simulink model "buck_discrete_sw_Close_Caso_2"  (R2025a)
settings: Solver=FixedStepDiscrete  StartTime=0.0  StopTime=inf  FixedStep=Tsim  RelTol=RelativeTolerance  EnableMultiTasking=on
undefined symbols (not defined in the file or in its folder): C_buck, DiscIntNeverNeededParam, L_buck, R, Scaling_Current, Scaling_Voltage, Vg
libraries: c2837xDlib x3
settings Model: ExtModeTrigDuration=8  Creator=Fernand  LastModifiedBy=Andres
settings DataIOCC: SaveFormat=StructureWithTime  ReturnWorkspaceOutputs=off  OutputSaveName=data_results  SignalLoggingName=DataResult
settings OptimizationCC: DefaultUnderspecifiedDataType=single  EnhancedBackFolding=on  PassReuseOutputArgsAs=Individual arguments  MaxStackSize=1024  OptimizeBlockOrder=speed  DifferentSizesBufferReuse=on  OptimizationCustomize=off  EfficientTunableParamExpr=on
settings DebuggingCC: ArtificialAlgebraicLoopMsg=none  ParameterTunabilityLossMsg=error
settings HardwareCC: ProdBitPerChar=16.0  ProdBitPerInt=16.0  ProdBitPerPointer=32.0  ProdBitPerSizeT=32.0  ProdBitPerPtrDiffT=32.0  ProdLargestAtomicInteger=Integer  ProdLargestAtomicFloat=None  ProdWordSize=16.0  ProdLongLongMode=on  ProdHWDeviceType=Texas Instruments->C2000  HardwareBoardFeatureSet=SoCBlockset
settings ModelReferenceCC: ModelReferenceNumInstancesAllowed=Single
settings SFSimCC: MATLABDynamicMemAlloc=off
settings RTWCC: SystemTargetFile=ert.tlc  HardwareBoard=TI Delfino F28379D LaunchPad  TemplateMakefile=ert_default_tmf  Toolchain=Texas Instruments Code Composer Studio (C2000)  CodeProfilingSaveOptions=MetricsOnly  GPUComputeCapability=3.5  Description=Embedded Coder
settings CodeAppCC: ForceParamTrailComments=on  IgnoreCustomStorageClasses=off  OperatorAnnotations=on  SimulinkDataObjDesc=on  SFDataObjDesc=on  InsertBlockDesc=on
settings ERTTargetCC: ExtModeTransport=4.0  ExtModeAutomaticAllocSize=off  ExtModeStaticAllocSize=10000.0  InlinedParameterPlacement=Hierarchical  DynamicArrayContainerType=coder::array  CodeReplacementLibrary=TI C28x  SubcomponentCodeInterfacePackaging=Nonreusable function  SupportContinuousTime=on

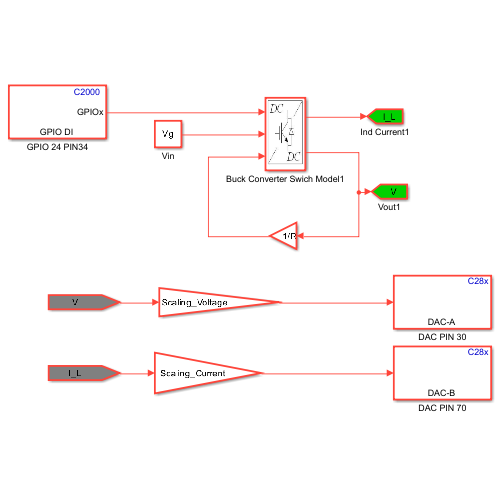
[thumbnail: Simulink's stored preview of the top-level diagram]
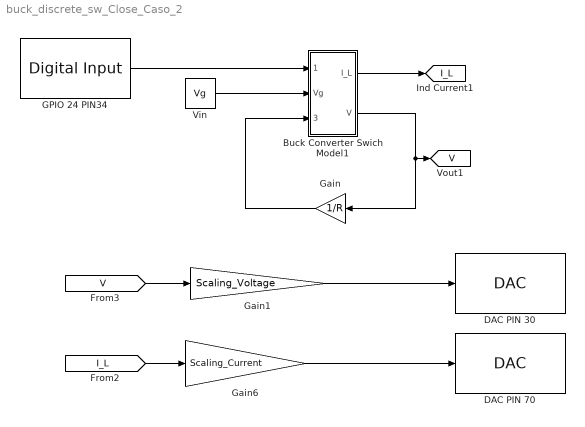
== system buck_discrete_sw_Close_Caso_2 ==
  Buck Converter Swich Model1 : Subsystem
      mask Display: image('$imagefile'); % Use "Edit Image" on toolstrip to change.
  DAC PIN 30 : c2837xDlib/DAC  channel=A  saturate=on
  DAC PIN 70 : c2837xDlib/DAC  channel=B  saturate=on
  GPIO 24 PIN34 : c2837xDlib/Digital Input  GPIO_Number=GPIO24~GPIO31  GPIO_Bit0=on  GPIO_Bit1=off  GPIO_Bit2=off  GPIO_Bit3=off  GPIO_Bit4=off  GPIO_Bit5=off  GPIO_Bit6=off  GPIO_Bit7=off  sampleTime=-1  dataType=auto  GPIO_Bit0_Qualification=Sync to SYSCLKOUT  GPIO_Bit1_Qualification=Sync to SYSCLKOUT  GPIO_Bit2_Qualification=Sync to SYSCLKOUT  GPIO_Bit3_Qualification=Sync to SYSCLKOUT  GPIO_Bit4_Qualification=Sync to SYSCLKOUT  GPIO_Bit5_Qualification=Sync to SYSCLKOUT  GPIO_Bit6_Qualification=Sync to SYSCLKOUT  GPIO_Bit7_Qualification=Sync to SYSCLKOUT  Qualification_Period=-1
  Gain : Gain  Gain=1/R
  Gain1 : Gain  Gain=Scaling_Voltage
  Gain6 : Gain  Gain=Scaling_Current
  Vin : Constant  Value=Vg  SampleTime=0
  tag scope: I_L=global, V=global
  wires:
  Vin/1 -> Buck Converter Swich Model1/2(Vg)
  Buck Converter Swich Model1/1(I_L) -> [I_L]
  Gain/1 -> Buck Converter Swich Model1/3(I_load)
  GPIO 24 PIN34/1 -> Buck Converter Swich Model1/1(PWM)
  Gain6/1 -> DAC PIN 70/1
  Gain1/1 -> DAC PIN 30/1
  [V] -> Gain1/1
  [I_L] -> Gain6/1
  Buck Converter Swich Model1/2(V) -> Gain/1, [V]

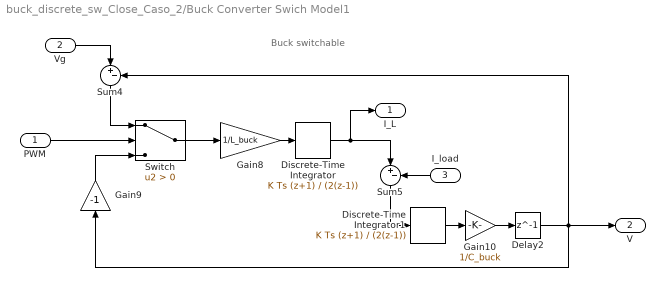
== system buck_discrete_sw_Close_Caso_2/Buck Converter Swich Model1 ==
  note: Buck switchable
  PWM : Inport
  Vg : Inport  Port=2
  I_load : Inport  Port=3
  Delay2 : Delay  DelayLength=1  InputProcessing=Columns as channels (frame based)
  Discrete-Time Integrator : DiscreteIntegrator  IntegratorMethod=Integration: Trapezoidal  SampleTime=-1  LimitOutput=on  LowerSaturationLimit=0  ICPrevOutput=DiscIntNeverNeededParam  ICPrevScaledInput=DiscIntNeverNeededParam
  Discrete-Time Integrator1 : DiscreteIntegrator  IntegratorMethod=Integration: Trapezoidal  SampleTime=-1  ICPrevOutput=DiscIntNeverNeededParam  ICPrevScaledInput=DiscIntNeverNeededParam
  Gain10 : Gain  Gain=1/C_buck
  Gain8 : Gain  Gain=1/L_buck
  Gain9 : Gain  Gain=-1
  Sum4 : Sum  Inputs=|+-
  Sum5 : Sum  Inputs=|+-
  Switch : Switch  Criteria=u2 > Threshold  SaturateOnIntegerOverflow=off  InputSameDT=off
  I_L : Outport
  V : Outport  Port=2
  wires:
  Gain9/1 -> Switch/3
  Switch/1 -> Gain8/1
  Sum4/1 -> Switch/1
  Gain8/1 -> Discrete-Time Integrator/1
  Sum5/1 -> Discrete-Time Integrator1/1
  Discrete-Time Integrator/1 -> I_L/1, Sum5/1
  Discrete-Time Integrator1/1 -> Gain10/1
  Vg/1 -> Sum4/1
  I_load/1 -> Sum5/2
  PWM/1 -> Switch/2
  Gain10/1 -> Delay2/1
  Delay2/1 -> Gain9/1, Sum4/2, V/1
